simulink model "variablearm"  (R2019b)
settings: Solver=VariableStepAuto  StartTime=0.0  StopTime=10  RelTol=1e-3
libraries: roblocks x4
settings Model: Creator=mads  LastModifiedBy=mads

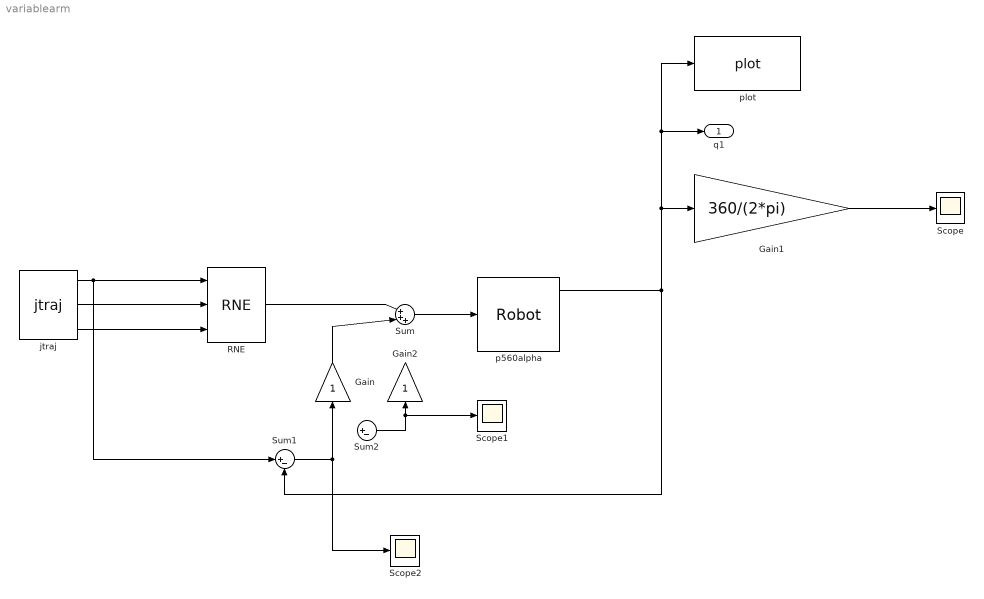
== system variablearm ==
  Gain : Gain
  Gain1 : Gain  Gain=360/(2*pi)
  Gain2 : Gain
  RNE : roblocks/Arm/RNE  robot=p560alpha  grav=[0 0 9.81]
  Scope : Scope
  Scope1 : Scope
  Scope2 : Scope
  Sum : Sum  Inputs=|+++
  Sum1 : Sum  Inputs=|+-
  Sum2 : Sum  Inputs=|+-
  jtraj : roblocks/Toolbox/jtraj  q0=[0 0 0]  qf=[pi/2 -pi/4 -pi/4]  tmax=2  ts=0.02
  p560alpha : roblocks/Arm/Robot  robot=p560alpha  q0=[0 0 0]
  plot : roblocks/Arm/plot  robot=p560alpha  fps=5  holdplot=on
  q1 : Outport  VectorParamsAs1DForOutWhenUnconnected=off
  wires:
  Gain1/1 -> Scope/1
  jtraj/1 -> Sum1/1, RNE/1
  jtraj/2 -> RNE/2
  jtraj/3 -> RNE/3
  RNE/1 -> Sum/1
  Sum/1 -> p560alpha/1
  Sum2/1 -> Scope1/1, Gain2/1
  p560alpha/1 -> plot/1, q1/1, Gain1/1, Sum1/2
  Sum1/1 -> Scope2/1, Gain/1
  Gain/1 -> Sum/2
